simulink model "TopDownTxRx"  (R2026a)
settings: Solver=VariableStepAuto  StopTime=inf  EnableMultiTasking=on
PreLoadFcn:
  | % Baseband parameters
  | bitRate = 250e3;
  | spf = 4;  % samples per frame
  | bps = 4;  % bits per ZigBee symbol
  | sps = 4;  % samples per OQPSK symbol
  | cps = 32;  % chips per ZigBee symbol
  | chipRate = bitRate * cps / bps;
  | 
  | % RF parameters
  | carrierFreqs = 2.45e9;  % Hz
  | harmonicOrder = 3;
  | oversampling = 1;  % no out-of-band signal
  | loToRFIsolation = inf;  % dB
  | demodIP2 = inf;  % dBm
  | 
  | % BER parameters
  | computationDelay = 0;
libraries: commdemoslib x2, TopDownRFReceiverDesignLib x2, commdigbbndpm3 x2, commrfcorlib x1, commrandsrc3 x1, simulink x1, commrflib2 x1, commsink2 x1, commutil2 x1, dspstat3 x1, dspmathops x1
Description:
  | Top-Down Design of Spread Spectrum Receiver for ZigBee
settings Model: Creator=The MathWorks, Inc.  LastModifiedBy=AYAN DAS
settings DebuggingCC: ConsistencyChecking=warning  UnderspecifiedInitializationDetection=Classic  MaxConsecutiveZCsMsg=warning
settings HardwareCC: ProdHWDeviceType=32-bit Generic
settings RTWCC: BuildConfiguration=Faster Runs
settings GRTTargetCC: CombineOutputUpdateFcns=off  GRTInterface=on
settings SimscapeCC: SimscapeNormalizeSystem=off  SimscapeNominalValues="[{\"value\":\"10\",\"unit\":\"V\"},{\"value\":\"1\",\"unit\":\"A\"},{\"value\":\"10\",\"unit\":\"N*m\"},{\"value\":\"10\",\"unit\":\"bar\"},{\"value\":\"100\",\"unit\":\"kJ/kg\"},{\"value\":\"1\",\"unit\":\"kW\"},{\"value\":\"300\",\"unit\":\"K\"},{\"value\":\"100\",\"unit\":\"cm^3/s\"},{\"value\":\"1\",\"unit\":\"kN\"},{\"value\":\"1\",\"unit\":\"g/cm^3\"},{\"value\":\"1\",\"unit\":\"l\"},{\"value\":\"1\",\"unit\":\"cm^2\"},{\"value\":\"60\",\"unit\":\"Hz\"}]"  SimscapeLogType=none  SimscapeLogDataHistory=5000.0

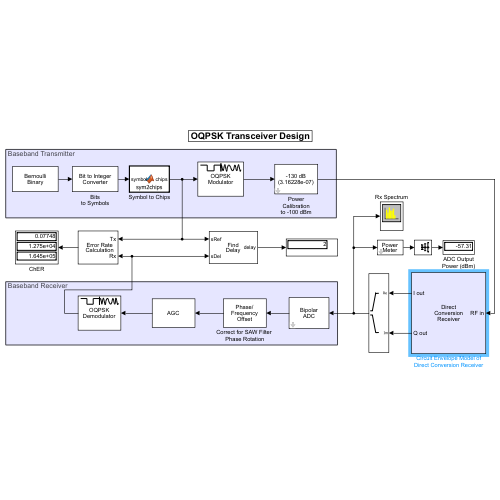
[thumbnail: Simulink's stored preview of the top-level diagram]
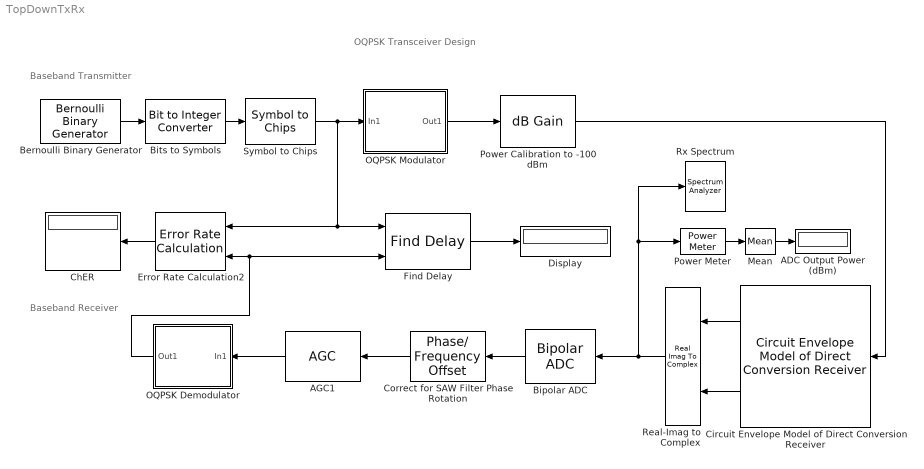
== system TopDownTxRx ==
  note: Baseband Transmitter
  note: Baseband Receiver
  note: OQPSK Transceiver Design
  ADC Output Power (dBm) : Display
  AGC1 : commrfcorlib/AGC  LegacyMode=off  DetectorMethod=Rectifier  LoopMethod=Linear  UpdatePeriod=100  StepSize=0.1  AdaptationStepSize=0.01  DesiredOutputPower=1  AveragingLength=100  MaximumGain=30  MaxPowerGain=200  GainOutputPort=off  InputPowerOutputPort=off  SimulateUsing=Interpreted execution
  Bernoulli Binary Generator : commrandsrc3/Bernoulli Binary Generator  ProbabilityOfZero=0.5  SeedSource=Parameter  Seed=73  SampleTime=1/bitRate  SamplesPerFrame=spf  OutputDataType=double  SimulateUsing=Interpreted execution
  Bipolar ADC : commdemoslib/Bipolar ADC  FS_V=0.0316  N=10
  Bits to Symbols : simulink/Logic and Bit Operations/Bit to Integer Converter  nbits=4  bitOrder=MSB first  signedOutputValues=Unsigned  outDtype=Inherit via internal rule  outDtypeSigned=Inherit via internal rule
  ChER : Display
  Circuit Envelope Model of Direct Conversion Receiver : TopDownRFReceiverDesignLib/Circuit Envelope Model of Direct Conversion Receiver  SystemSampleTime=-1  VariantActivationTime=update diagram  EmptyChoice=off  PassThrough=off  PassThroughVariantControl=(default)  EmptyChoiceVariantControl=(default)  AllowFlexibleInterface=on  Latency=0  AutoFrameSizeCalculation=off
  Correct for SAW Filter Phase Rotation : commrflib2/Phase// Frequency Offset  PhaseOffset=58  FrequencyOffsetFromPort=off  FrequencyOffset=0  SimulateUsing=Code generation
  Display : Display
  Error Rate Calculation2 : commsink2/Error Rate Calculation  N="2  % Demod delay, half the filter length"  st_delay=computationDelay  cp_mode=Entire frame  subframe=[]  PMode=Port  WsName=ErrorVec  RsMode2=off  stop=off  numErr=2e3  maxBits=1e7
  Find Delay : commutil2/Find Delay  corrLength=200  chgSigOP=off  stopUpdate=off  numConstDelay=3
  Mean : dspstat3/Mean  run=on  InputProcessing=Columns as channels (frame based)  reset_popup=None  directionMode=Each column  dimension=1  roiEnable=off  roiType=Rectangles  roiPortion=Entire ROI  roiOutput=Individual statistics for each ROI  roiFlag=off  roundingMode=Floor  overflowMode=off  outputDataTypeStr=Inherit: Same as accumulator  outputMin=[]  outputMax=[]  outputLastDataTypeStr=Inherit: Same as accumulator
  OQPSK Demodulator : Subsystem
      mask Display:
      | plot(0,0,100,100,[5+15*[0 1 1 2 2 3] 50 50 50 50+1.5*[[0:.8:10] [10:1.6:20] [20:.8:30]]],[85+8*[1 1 -1 -1 1 1] 85 99 75 85+10*[sin([0:.8:10]*pi*2/5) sin([10:1.6:20]*pi/5) sin([20:.8:30]*pi*2/5)]]);
      | disp('OQPSK\nDemodulator')
  "OQPSK Modulator " : Subsystem
      mask Display:
      | plot(0,0,100,100,[5+15*[0 1 1 2 2 3] 50 50 50 50+1.5*[[0:.8:10] [10:1.6:20] [20:.8:30]]],[85+8*[1 1 -1 -1 1 1] 85 99 75 85+10*[sin([0:.8:10]*pi*2/5) sin([10:1.6:20]*pi/5) sin([20:.8:30]*pi*2/5)]]);
      | disp('OQPSK\nModulator')
  Power Calibration to -100 dBm : dspmathops/dB Gain  dB="-130  % power of preceding block is 1 W"  intype=Amplitude
  Power Meter : commdemoslib/Power Meter  R=1  N=1024
  Real-Imag to Complex : RealImagToComplex
  Rx Spectrum : SpectrumAnalyzer  WindowPosition=[280.000000,112.000000,721.000000,496.000000,]  Visible=on  ScopeFrameLocation=window  SampleRate=4000000  AxesScaling=Manual  FrequencyResolutionMethod=Window length  RBWSource=Property  RBW=46921.92192  FFTLength=128  Span=32000000  StartFrequency=-16000000  StopFrequency=16000000  AveragingMethod=Running  SpectralAverages=2000  ForgettingFactor=0.99  FrequencyOffset=2.45e9  MaximizeAxes=Off  YLabel=Power  YLimits=[-102.64356838478707 -35.77608892868329]  AllowFFTLengthLessThanSamplesPerUpdate=on  DefaultConfigurationName=spbscopes.SpectrumAnalyzerBlockCfg  IsFrequencyInputMode=0  FrequencyVectorPort=0  FrequencyVectorFromPort=0  FrequencyInputRBWPort=0  FrequencyInputRBWFromPort=0  SegLen=1024
  Symbol to Chips : TopDownRFReceiverDesignLib/802.15 Transmitter/Symbol to Chips  SystemSampleTime=-1  VariantActivationTime=update diagram  EmptyChoice=off  PassThrough=off  PassThroughVariantControl=(default)  EmptyChoiceVariantControl=(default)  AllowFlexibleInterface=on  Latency=0  AutoFrameSizeCalculation=off
  wires:
  Bits to Symbols/1 -> Symbol to Chips/1
  Power Calibration to -100 dBm/1 -> Circuit Envelope Model of Direct Conversion Receiver/1
  Bernoulli Binary Generator/1 -> Bits to Symbols/1
  Error Rate Calculation2/1 -> ChER/1
  Correct for SAW Filter Phase Rotation/1 -> AGC1/1
  OQPSK Demodulator/1(Out1) -> Find Delay/2, Error Rate Calculation2/2
  Bipolar ADC/1 -> Correct for SAW Filter Phase Rotation/1
  Mean/1 -> ADC Output Power (dBm)/1
  Power Meter/1 -> Mean/1
  Real-Imag to Complex/1 -> Bipolar ADC/1, Rx Spectrum/1, Power Meter/1
  Circuit Envelope Model of Direct Conversion Receiver/1 -> Real-Imag to Complex/1
  Circuit Envelope Model of Direct Conversion Receiver/2 -> Real-Imag to Complex/2
  Symbol to Chips/1 -> "OQPSK Modulator "/1(In1), Error Rate Calculation2/1, Find Delay/1
  "OQPSK Modulator "/1(Out1) -> Power Calibration to -100 dBm/1
  AGC1/1 -> OQPSK Demodulator/1(In1)
  Find Delay/1 -> Display/1

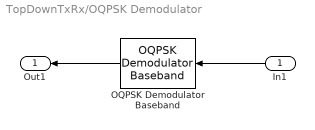
== system TopDownTxRx/OQPSK Demodulator ==
  In1 : Inport
  OQPSK Demodulator Baseband : commdigbbndpm3/OQPSK Demodulator Baseband  OutType=Bit  Ph=0  Mapping=Gray  pulseShape=Half sine  num=[0.7071, 0.7071]  rolloff=0.2  filterSpan=10  sps=sps  RateOptions=Enforce single-rate processing  outDtype2=double
  Out1 : Outport
  wires:
  OQPSK Demodulator Baseband/1 -> Out1/1
  In1/1 -> OQPSK Demodulator Baseband/1

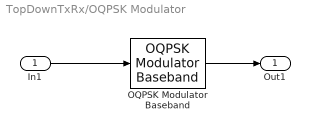
== system TopDownTxRx/OQPSK Modulator  ==
  In1 : Inport
  OQPSK Modulator Baseband : commdigbbndpm3/OQPSK Modulator Baseband  VariantControl=strcmp(pulseShape, 'Custom') && isequal(denom, 1)  InType=Bit  Mapping=Gray  Ph=0  pulseShape=Half sine  num=[0.7071, 0.7071]  denom=[1]  rolloff=0.2  filterSpan=10  sps=sps  RateOptions=Enforce single-rate processing  outDtype=double  isIIR=off
  Out1 : Outport
  wires:
  In1/1 -> OQPSK Modulator Baseband/1
  OQPSK Modulator Baseband/1 -> Out1/1
